simulink library "adrcLibrary"  (R2021a)
settings: Solver=VariableStepAuto  StartTime=0.0  StopTime=10.0  RelTol=1e-3
undefined symbols (not defined in the file or in its folder): DiscIntNeverNeededParam, r0
settings Model: Creator=onqi  LastModifiedBy=onqi

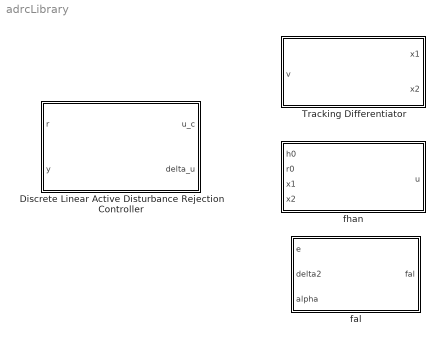
== system adrcLibrary ==
  Discrete Linear Active Disturbance Rejection Controller : Subsystem  Variant=on  VariantControl=Choice  mask(Linear Active Disturbance Rejection Control){order=1, b0=1, w_cl=1, k_eso=1, eso_init=[0;0], m_lim=[-inf, inf], r_lim=[-inf, inf], halfgain_ctrl=off, halfgain_obsv=off, inc_form=on, SampleTime=-1}
      mask prompts: order "First- or second-order ADRC"; b0 "Gain parameter b0"; w_cl "Desired closed-loop bandwidth w_cl [rad/s]"; k_eso "Relational observer bandwidth k_eso"; eso_init "Initial state of extended state observer"; m_lim "Magnitude limit of controller [lo, hi]"; r_lim "Rate limit of controller [lo, hi]"; halfgain_ctrl "Toggle half-gain tuning for controller"; halfgain_obsv "Toggle half-gain tuning for observer"; inc_form "Incremental form of ADRC"; SampleTime "Simulink:blkprm_prompts:AllBlksSampleTime"
      mask help:
      | Linear Active Disturbance Rejection Control block implementing the algorithms described in
      |
      | - Practical Active Disturbance Rejection Control: Bumpless Transfer, Rate Limitation and Incremental Algorithm, Gernot Herbst
      | - Half-Gain Tuning for Active Disturbance Rejection Control, Herbst et al.
      mask init:
      | ADRC_INC_FORM = inc_form;
      | 
      | if order == 1
      |     Ad = [[1, SampleTime];[0, 1]];
      |     Bd = [b0 * SampleTime; 0];
      |     Cd = [1, 0];
      |     Dd = 0;
      |     % Controller parameters for closed-loop dynamics
      |     t_settle = 4 / w_cl;
      |     sCL = -4 / t_settle;
      |     Kp = -2 * sCL;
      |     % Observer dynamics
      |     sESO = k_eso * sCL;
      |     zESO = exp(sESO * SampleTime);
      | 
      |     % Observer gains resulting in common-location observer poles
      |     L = [1 - zESO^2; (1 / SampleTime) * (1 - zESO)^2];
      | 
      |     % Controller gains
      |     w = [Kp / b0; 1 / b0];
      | 
      | elseif order == 2
      |     Ad = [[1, SampleTime, (SampleTime^2) / 2]; [0, 1, SampleTime]; [0, 0, 1]];
      |     Bd = [b0 * (SampleTime^2) / 2; b0 * SampleTime; 0];
      |     Cd = [1, 0, 0];
      |     Dd = 0;
      | 
      |     % Controller parameters for closed-loop dynamics
      |     t_settle = 6 / w_cl;
      |     sCL = -6 / t_settle;
      |     Kp = sCL^2;
      |     Kd = -2 * sCL;
      | 
      |     % Observer dynamics
      |     sESO = k_eso * sCL;
      |     zESO = exp(sESO * SampleTime);
      | 
      |     % Observer gains resulting in common-location observer poles
      |     L = [1 - (zESO)^3; (3 / (2 * SampleTime)) * (1 - zESO)^2 * (1 + zESO); 
      |         (1 / SampleTime^2) * (1 - zESO)^3];
      | 
      |     % Controller gains
      |     w = [Kp / b0; Kd / b0; 1 / b0];
      | end
      | 
      | if halfgain_obsv
      |     L = L/2;
      | end
      | 
      | if halfgain_ctrl
      |     w = w/2;
      | end
      | 
      | % One-step update equation implementing linear ESO
      | A_ESO = Ad - L * Cd * Ad;
      | B_ESO = Bd - L * Cd * Bd;
      | C_ESO = Cd;
      | 
      | L_ESO = L;
      settings: CopyFcn=set_param(gcbh,'LinkStatus','none');
      mask TypeOptions order: 1 | 2
      mask TypeOptions SampleTime: r/SampleTime
      mask DialogControl SampleTime Prompt: Sample time (-1 for inherited):
      mask Display:
      | disp('Discrete Linear\nADRC');
      | 
      | port_label('output', 1, 'u[k]', 'texmode', 'on');
      | port_label('input', 2, 'y[k-1]', 'texmode', 'on');
      | port_label('input', 1, 'r[k]', 'texmode', 'on');
      | 
      | if ADRC_INC_FORM == 1
      |     port_label('output', 2, '\Deltau', 'texmode', 'on');
      | end
  Tracking Differentiator : Subsystem  SystemSampleTime=SystemSampleTime  mask{r0=50, h0=10, SystemSampleTime=-1}
      mask prompts: r0 "Tracking speed r0"; h0 "Tracking smoothness h0"; SystemSampleTime "Simulink:blkprm_prompts:AllBlksSampleTime"
      mask init:
      | h = str2num(get_param(gcs,'FixedStep'));
      mask TypeOptions SystemSampleTime: SystemSampleTime
      mask DialogControl SystemSampleTime Prompt: Sample time (-1 for inherited):
      mask Display:
      | disp('Tracking Differentiator')
      | port_label('input', 1, '\vee', 'texmode', 'on');
      | port_label('output', 1, 'x_1', 'texmode', 'on');
      | port_label('output', 2, '\Deltax_1', 'texmode', 'on');
  fal : Subsystem
      mask Display:
      | disp('fal(e, \alpha, \delta)', 'texmode', 'on')
      | port_label('input', 1, 'e', 'texmode', 'on');
      | port_label('output', 1, 'fal', 'texmode', 'on');
      | port_label('input', 2, '\delta', 'texmode', 'on');
      | port_label('input', 3, '\alpha', 'texmode', 'on');
  fhan : Subsystem
      mask Display:
      | disp('fhan(x_1, x_2, r, h)', 'texmode', 'on')
      | port_label('input', 1, 'h_0', 'texmode', 'on');
      | port_label('input', 2, 'r_0', 'texmode', 'on');
      | port_label('input', 3, 'x_1', 'texmode', 'on');
      | port_label('input', 4, 'x_2', 'texmode', 'on');
      | 
      | port_label('output', 1, 'f_{han}', 'texmode', 'on');

== system adrcLibrary/Discrete Linear Active Disturbance Rejection Controller ==
  r : Inport  SampleTime=SampleTime
  y : Inport  Port=2
  Incremental Form : Subsystem  VariantControl=inc_form == 1
  Non-Incremental Form : Subsystem  VariantControl=inc_form == 0
  u_c : Outport
  delta_u : Outport  Port=2

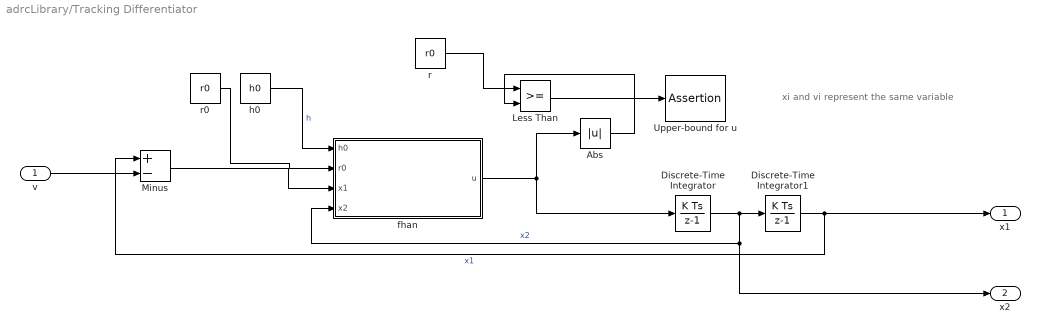
== system adrcLibrary/Tracking Differentiator ==
  note: xi and vi represent the same variable
  v : Inport
  Abs : Abs
  Discrete-Time Integrator : DiscreteIntegrator  SampleTime=-1  ICPrevOutput=DiscIntNeverNeededParam  ICPrevScaledInput=DiscIntNeverNeededParam
  Discrete-Time Integrator1 : DiscreteIntegrator  SampleTime=-1  ICPrevOutput=DiscIntNeverNeededParam  ICPrevScaledInput=DiscIntNeverNeededParam
  Less Than : RelationalOperator  OutDataTypeStr=boolean  RndMeth=Simplest
  Minus : Sum  Inputs=+-
  Upper-bound for u : Assertion
  fhan : Subsystem
  h0 : Constant  Value=h0  SampleTime=-1
  r : Constant  Value=r0  SampleTime=-1
  r0 : Constant  Value=r0  SampleTime=-1
  x1 : Outport
  x2 : Outport  Port=2
  wires:
  Abs/1 -> Less Than/2
  Less Than/1 -> Upper-bound for u/1
  Discrete-Time Integrator1/1 -> x1/1, Minus/1  "x1"
  Discrete-Time Integrator/1 -> fhan/4(x2), x2/1, Discrete-Time Integrator1/1  "x2"
  v/1 -> Minus/2
  r/1 -> Less Than/1
  fhan/1(u) -> Discrete-Time Integrator/1, Abs/1
  h0/1 -> fhan/1(h0)  "h"
  r0/1 -> fhan/2(r0)
  Minus/1 -> fhan/3(x1)

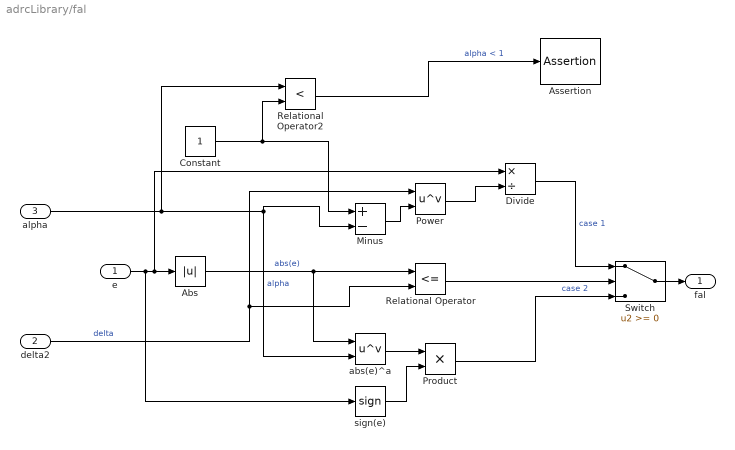
== system adrcLibrary/fal ==
  e : Inport
  delta2 : Inport  Port=2
  alpha : Inport  Port=3
  Abs : Abs
  Assertion : Assertion
  Constant : Constant
  Divide : Product  Inputs=*/
  Minus : Sum  Inputs=+-
  Power : Math  Operator=pow  SaturateOnIntegerOverflow=on
  Product : Product
  Relational Operator : RelationalOperator  Operator=<=  OutDataTypeStr=boolean  RndMeth=Simplest
  Relational Operator2 : RelationalOperator  Operator=<  OutDataTypeStr=boolean  RndMeth=Simplest
  Switch : Switch
  abs(e)^a : Math  Operator=pow  SaturateOnIntegerOverflow=on
  sign(e) : Signum
  fal : Outport
  wires:
  sign(e)/1 -> Product/2
  Switch/1 -> fal/1
  Relational Operator/1 -> Switch/2
  Abs/1 -> abs(e)^a/1, Relational Operator/1  "abs(e)"
  Power/1 -> Divide/2
  alpha/1 -> Relational Operator2/1, Minus/2, abs(e)^a/2  "alpha"
  Minus/1 -> Power/2
  e/1 -> sign(e)/1, Divide/1, Abs/1
  abs(e)^a/1 -> Product/1
  Product/1 -> Switch/3  "case 2"
  Divide/1 -> Switch/1  "case 1"
  delta2/1 -> Relational Operator/2, Power/1  "delta"
  Constant/1 -> Relational Operator2/2, Minus/1
  Relational Operator2/1 -> Assertion/1  "alpha < 1"

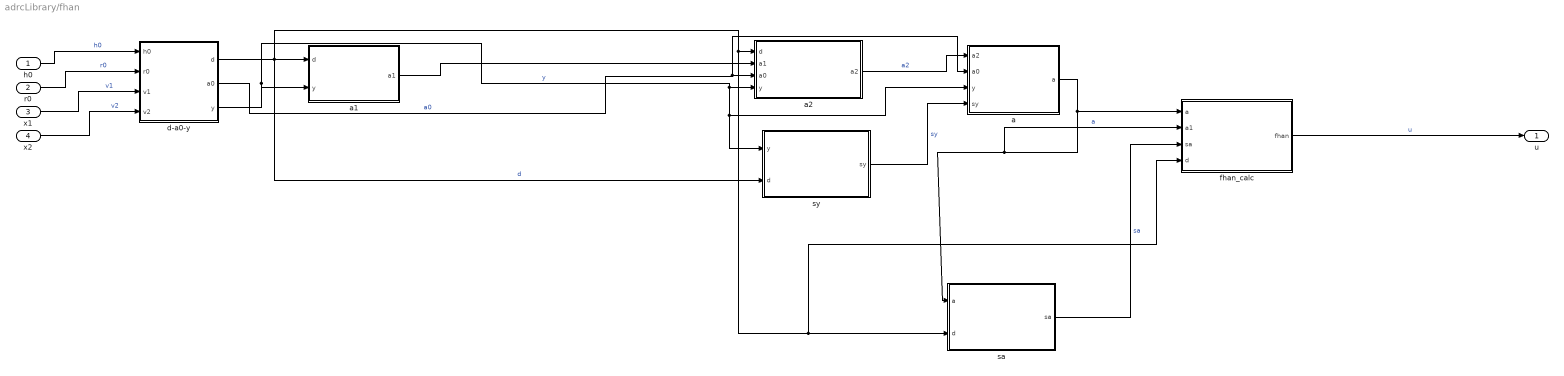
== system adrcLibrary/fhan ==
  h0 : Inport
  r0 : Inport  Port=2
  x1 : Inport  Port=3
  x2 : Inport  Port=4
  a : Subsystem
  a1 : Subsystem
  a2 : Subsystem
  d-a0-y : Subsystem
  fhan_calc : Subsystem
  sa : Subsystem
  sy : Subsystem
  u : Outport
  wires:
  h0/1 -> d-a0-y/1(h0)  "h0"
  r0/1 -> d-a0-y/2(r0)  "r0"
  x1/1 -> d-a0-y/3(v1)  "v1"
  x2/1 -> d-a0-y/4(v2)  "v2"
  d-a0-y/1(d) -> sy/2(d), a1/1(d), fhan_calc/4(d), sa/2(d), a2/1(d)  "d"
  d-a0-y/3(y) -> a/3(y), sy/1(y), a2/4(y), a1/2(y)  "y"
  a1/1(a1) -> a2/2(a1)
  d-a0-y/2(a0) -> a/2(a0), a2/3(a0)  "a0"
  a2/1(a2) -> a/1(a2)  "a2"
  sy/1(sy) -> a/4(sy)  "sy"
  a/1(a) -> sa/1(a), fhan_calc/2(a1), fhan_calc/1(a)  "a"
  sa/1(sa) -> fhan_calc/3(sa)  "sa"
  fhan_calc/1(fhan) -> u/1  "u"

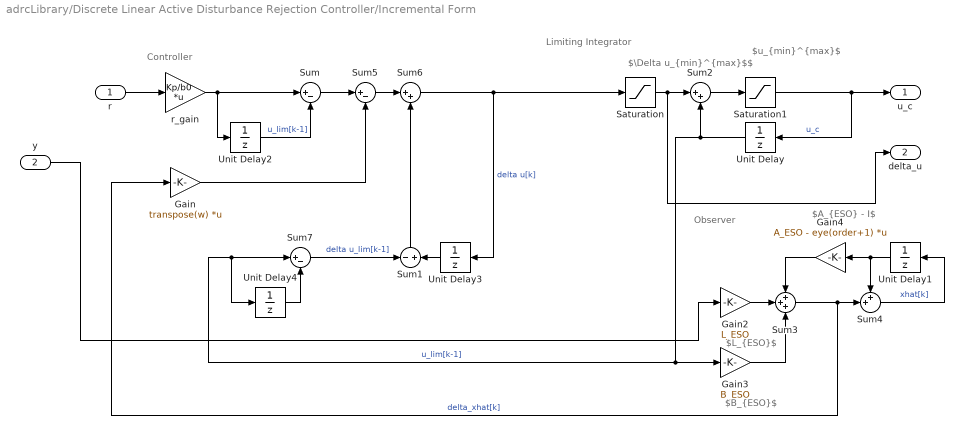
== system adrcLibrary/Discrete Linear Active Disturbance Rejection Controller/Incremental Form ==
  note: Controller
  note: $\Delta u_{min}^{max}$$
  note: $u_{min}^{max}$
  note: $L_{ESO}$
  note: $B_{ESO}$
  note: $A_{ESO} - I$
  note: Limiting
      | 	Integrator
  note: Observer
  r : Inport  SampleTime=SampleTime
  y : Inport  Port=2
  Gain : Gain  Gain=transpose(w)  Multiplication=Matrix(K*u) (u vector)
  Gain2 : Gain  Gain=L_ESO
  Gain3 : Gain  Gain=B_ESO
  Gain4 : Gain  Gain=A_ESO - eye(order+1)  Multiplication=Matrix(K*u) (u vector)
  Saturation : Saturate  UpperLimit=r_lim(2)  LowerLimit=r_lim(1)
  Saturation1 : Saturate  UpperLimit=m_lim(2)  LowerLimit=m_lim(1)
  Sum : Sum  Inputs=|+-
  Sum1 : Sum  Inputs=-+
  Sum2 : Sum  Inputs=|++
  Sum3 : Sum  Inputs=+++
  Sum4 : Sum  Inputs=++|
  Sum5 : Sum  Inputs=|+-
  Sum6 : Sum  Inputs=|++
  Sum7 : Sum  Inputs=|+-
  Unit Delay{,1..4} (5 alike) : UnitDelay  SampleTime=-1  HasFrameUpgradeWarning=on
  r_gain : Gain  Gain=Kp/b0  Multiplication=Matrix(K*u) (u vector)
  u_c : Outport
  delta_u : Outport  Port=2
  wires:
  Unit Delay1/1 -> Sum4/1, Gain4/1
  Sum2/1 -> Saturation1/1
  Gain4/1 -> Sum3/1
  Gain3/1 -> Sum3/3
  y/1 -> Gain2/1
  Sum6/1 -> Unit Delay3/1, Saturation/1  "delta u[k]"
  Saturation1/1 -> u_c/1, Unit Delay/1  "u_c"
  Unit Delay/1 -> Gain3/1, Unit Delay4/1, Sum7/1, Sum2/2  "u_lim[k-1]"
  Saturation/1 -> delta_u/1, Sum2/1
  r_gain/1 -> Unit Delay2/1, Sum/1
  r/1 -> r_gain/1
  Gain2/1 -> Sum3/2
  Sum4/1 -> Unit Delay1/1  "xhat[k]"
  Sum3/1 -> Gain/1, Sum4/2  "delta_xhat[k]"
  Sum/1 -> Sum5/1
  Sum5/1 -> Sum6/1
  Unit Delay2/1 -> Sum/2  "u_lim[k-1]"
  Gain/1 -> Sum5/2
  Unit Delay3/1 -> Sum1/2
  Sum1/1 -> Sum6/2
  Sum7/1 -> Sum1/1  "delta u_lim[k-1]"
  Unit Delay4/1 -> Sum7/2

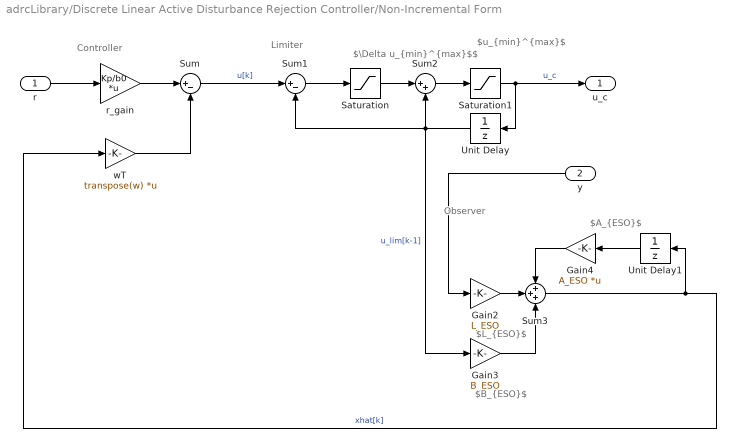
== system adrcLibrary/Discrete Linear Active Disturbance Rejection Controller/Non-Incremental Form ==
  note: Controller
  note: $\Delta u_{min}^{max}$$
  note: $u_{min}^{max}$
  note: $L_{ESO}$
  note: $B_{ESO}$
  note: $A_{ESO}$
  note: Limiter
  note: Observer
  r : Inport  SampleTime=SampleTime
  y : Inport  Port=2
  Gain2 : Gain  Gain=L_ESO
  Gain3 : Gain  Gain=B_ESO
  Gain4 : Gain  Gain=A_ESO  Multiplication=Matrix(K*u) (u vector)
  Saturation : Saturate  UpperLimit=r_lim(2)  LowerLimit=r_lim(1)
  Saturation1 : Saturate  UpperLimit=m_lim(2)  LowerLimit=m_lim(1)
  Sum : Sum  Inputs=|+-
  Sum1 : Sum  Inputs=|+-
  Sum2 : Sum  Inputs=|++
  Sum3 : Sum  Inputs=+++
  Unit Delay : UnitDelay  SampleTime=-1  HasFrameUpgradeWarning=on
  Unit Delay1 : UnitDelay  SampleTime=-1  HasFrameUpgradeWarning=on
  r_gain : Gain  Gain=Kp/b0  Multiplication=Matrix(K*u) (u vector)
  wT : Gain  Gain=transpose(w)  Multiplication=Matrix(K*u) (u vector)
  u_c : Outport
  wires:
  Unit Delay1/1 -> Gain4/1
  wT/1 -> Sum/2
  Sum2/1 -> Saturation1/1
  Gain4/1 -> Sum3/1
  Gain3/1 -> Sum3/3
  y/1 -> Gain2/1
  Sum1/1 -> Saturation/1
  Saturation1/1 -> u_c/1, Unit Delay/1  "u_c"
  Unit Delay/1 -> Gain3/1, Sum2/2, Sum1/2  "u_lim[k-1]"
  Saturation/1 -> Sum2/1
  r_gain/1 -> Sum/1
  r/1 -> r_gain/1
  Sum/1 -> Sum1/1  "u[k]"
  Sum3/1 -> wT/1, Unit Delay1/1  "xhat[k]"
  Gain2/1 -> Sum3/2

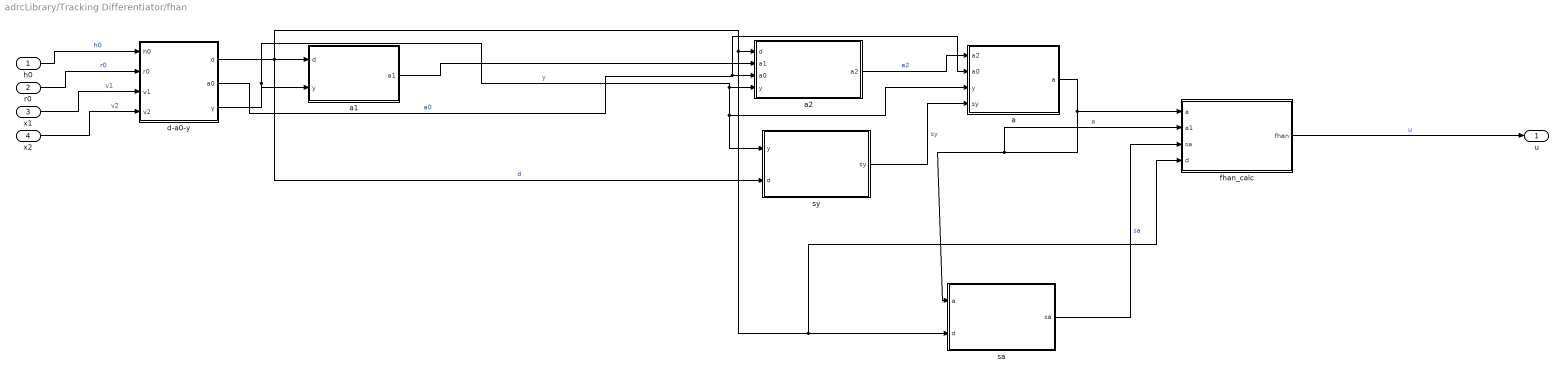
== system adrcLibrary/Tracking Differentiator/fhan ==
  h0 : Inport
  r0 : Inport  Port=2
  x1 : Inport  Port=3
  x2 : Inport  Port=4
  a : Subsystem
  a1 : Subsystem
  a2 : Subsystem
  d-a0-y : Subsystem
  fhan_calc : Subsystem
  sa : Subsystem
  sy : Subsystem
  u : Outport
  wires:
  h0/1 -> d-a0-y/1(h0)  "h0"
  r0/1 -> d-a0-y/2(r0)  "r0"
  x1/1 -> d-a0-y/3(v1)  "v1"
  x2/1 -> d-a0-y/4(v2)  "v2"
  d-a0-y/1(d) -> sy/2(d), a1/1(d), fhan_calc/4(d), sa/2(d), a2/1(d)  "d"
  d-a0-y/3(y) -> a/3(y), sy/1(y), a2/4(y), a1/2(y)  "y"
  a1/1(a1) -> a2/2(a1)
  d-a0-y/2(a0) -> a/2(a0), a2/3(a0)  "a0"
  a2/1(a2) -> a/1(a2)  "a2"
  sy/1(sy) -> a/4(sy)  "sy"
  a/1(a) -> sa/1(a), fhan_calc/2(a1), fhan_calc/1(a)  "a"
  sa/1(sa) -> fhan_calc/3(sa)  "sa"
  fhan_calc/1(fhan) -> u/1  "u"

== system adrcLibrary/fhan/a ==
  a2 : Inport
  a0 : Inport  Port=2
  y : Inport  Port=3
  sy : Inport  Port=4
  Add : Sum  Inputs=++-
  Plus : Sum
  Product : Product
  a : Outport
  wires:
  y/1 -> Add/2
  a0/1 -> Add/1
  Plus/1 -> a/1  "a"
  a2/1 -> Plus/2, Add/3
  Product/1 -> Plus/1
  sy/1 -> Product/2
  Add/1 -> Product/1

== system adrcLibrary/fhan/a1 ==
  d : Inport
  y : Inport  Port=2
  Abs : Abs
  Add : Sum
  Gain : Gain  Gain=8
  Product : Product
  Sqrt : Sqrt  SaturateOnIntegerOverflow=on
  a1 : Outport
  wires:
  Product/1 -> Sqrt/1
  Sqrt/1 -> a1/1  "a1"
  y/1 -> Abs/1
  d/1 -> Product/1, Add/1
  Add/1 -> Product/2
  Abs/1 -> Gain/1
  Gain/1 -> Add/2  "8|y|"

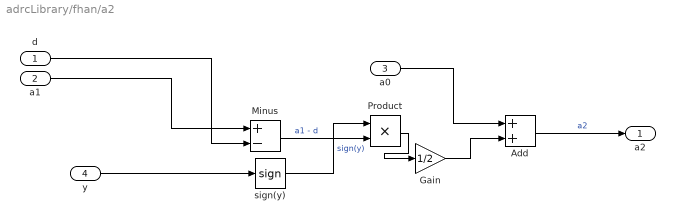
== system adrcLibrary/fhan/a2 ==
  d : Inport
  a1 : Inport  Port=2
  a0 : Inport  Port=3
  y : Inport  Port=4
  Add : Sum
  Gain : Gain  Gain=1/2
  Minus : Sum  Inputs=+-
  Product : Product
  sign(y) : Signum
  a2 : Outport
  wires:
  sign(y)/1 -> Product/1  "sign(y)"
  Minus/1 -> Product/2  "a1 - d"
  Product/1 -> Gain/1
  y/1 -> sign(y)/1
  a0/1 -> Add/1
  d/1 -> Minus/2
  Add/1 -> a2/1  "a2"
  a1/1 -> Minus/1
  Gain/1 -> Add/2

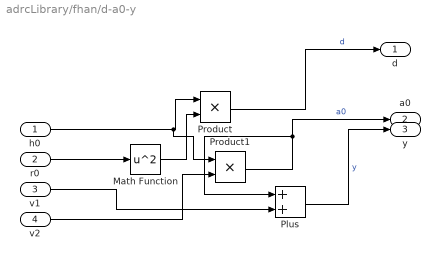
== system adrcLibrary/fhan/d-a0-y ==
  h0 : Inport
  r0 : Inport  Port=2
  v1 : Inport  Port=3
  v2 : Inport  Port=4
  Math Function : Math  Operator=square  SaturateOnIntegerOverflow=on
  Plus : Sum
  Product : Product
  Product1 : Product
  d : Outport
  a0 : Outport  Port=2
  y : Outport  Port=3
  wires:
  Math Function/1 -> Product/2
  v1/1 -> Plus/2
  Plus/1 -> y/1  "y"
  r0/1 -> Math Function/1
  Product1/1 -> a0/1, Plus/1  "a0"
  v2/1 -> Product1/2
  Product/1 -> d/1  "d"
  h0/1 -> Product1/1, Product/1

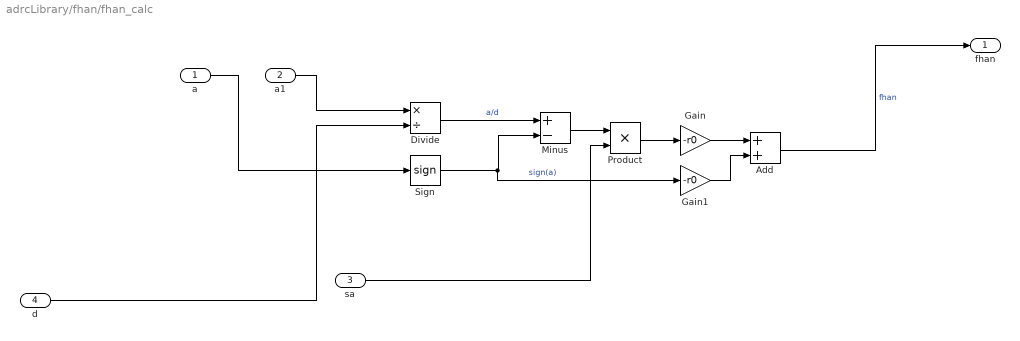
== system adrcLibrary/fhan/fhan_calc ==
  a : Inport
  a1 : Inport  Port=2
  sa : Inport  Port=3
  d : Inport  Port=4
  Add : Sum
  Divide : Product  Inputs=*/
  Gain : Gain  Gain=-r0
  Gain1 : Gain  Gain=-r0
  Minus : Sum  Inputs=+-
  Product : Product
  Sign : Signum
  fhan : Outport
  wires:
  sa/1 -> Product/2
  Minus/1 -> Product/1
  Gain/1 -> Add/1
  Divide/1 -> Minus/1  "a/d"
  a/1 -> Sign/1
  Add/1 -> fhan/1  "fhan"
  a1/1 -> Divide/1
  Gain1/1 -> Add/2
  d/1 -> Divide/2
  Product/1 -> Gain/1
  Sign/1 -> Gain1/1, Minus/2  "sign(a)"

== system adrcLibrary/fhan/sa ==
  a : Inport
  d : Inport  Port=2
  Gain : Gain  Gain=1/2
  Minus : Sum  Inputs=+-
  Minus1 : Sum  Inputs=+-
  Plus : Sum
  Sign1 : Signum
  Sign2 : Signum
  sa : Outport
  wires:
  Sign1/1 -> Minus1/1
  Plus/1 -> Sign1/1
  a/1 -> Minus/1, Plus/1
  Sign2/1 -> Minus1/2
  Minus/1 -> Sign2/1
  Minus1/1 -> Gain/1
  d/1 -> Minus/2, Plus/2
  Gain/1 -> sa/1  "s"

== system adrcLibrary/fhan/sy ==
  y : Inport
  d : Inport  Port=2
  Gain : Gain  Gain=1/2
  Minus : Sum  Inputs=+-
  Minus1 : Sum  Inputs=+-
  Plus : Sum
  Sign1 : Signum
  Sign2 : Signum
  sy : Outport
  wires:
  Sign1/1 -> Minus1/1
  Plus/1 -> Sign1/1
  y/1 -> Minus/1, Plus/1
  Sign2/1 -> Minus1/2
  Minus/1 -> Sign2/1
  Minus1/1 -> Gain/1
  d/1 -> Minus/2, Plus/2
  Gain/1 -> sy/1  "s"

== system adrcLibrary/Tracking Differentiator/fhan/a ==
  a2 : Inport
  a0 : Inport  Port=2
  y : Inport  Port=3
  sy : Inport  Port=4
  Add : Sum  Inputs=++-
  Plus : Sum
  Product : Product
  a : Outport
  wires:
  y/1 -> Add/2
  a0/1 -> Add/1
  Plus/1 -> a/1  "a"
  a2/1 -> Plus/2, Add/3
  Product/1 -> Plus/1
  sy/1 -> Product/2
  Add/1 -> Product/1

== system adrcLibrary/Tracking Differentiator/fhan/a1 ==
  d : Inport
  y : Inport  Port=2
  Abs : Abs
  Add : Sum
  Gain : Gain  Gain=8
  Product : Product
  Sqrt : Sqrt  SaturateOnIntegerOverflow=on
  a1 : Outport
  wires:
  Product/1 -> Sqrt/1
  Sqrt/1 -> a1/1  "a1"
  y/1 -> Abs/1
  d/1 -> Product/1, Add/1
  Add/1 -> Product/2
  Abs/1 -> Gain/1
  Gain/1 -> Add/2  "8|y|"

== system adrcLibrary/Tracking Differentiator/fhan/a2 ==
  d : Inport
  a1 : Inport  Port=2
  a0 : Inport  Port=3
  y : Inport  Port=4
  Add : Sum
  Gain : Gain  Gain=1/2
  Minus : Sum  Inputs=+-
  Product : Product
  sign(y) : Signum
  a2 : Outport
  wires:
  sign(y)/1 -> Product/1  "sign(y)"
  Minus/1 -> Product/2  "a1 - d"
  Product/1 -> Gain/1
  y/1 -> sign(y)/1
  a0/1 -> Add/1
  d/1 -> Minus/2
  Add/1 -> a2/1  "a2"
  a1/1 -> Minus/1
  Gain/1 -> Add/2

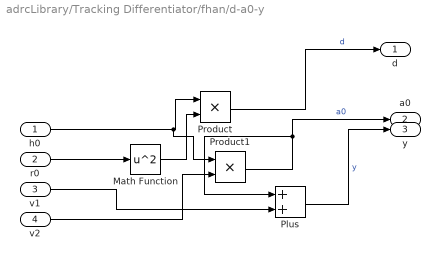
== system adrcLibrary/Tracking Differentiator/fhan/d-a0-y ==
  h0 : Inport
  r0 : Inport  Port=2
  v1 : Inport  Port=3
  v2 : Inport  Port=4
  Math Function : Math  Operator=square  SaturateOnIntegerOverflow=on
  Plus : Sum
  Product : Product
  Product1 : Product
  d : Outport
  a0 : Outport  Port=2
  y : Outport  Port=3
  wires:
  Math Function/1 -> Product/2
  v1/1 -> Plus/2
  Plus/1 -> y/1  "y"
  r0/1 -> Math Function/1
  Product1/1 -> a0/1, Plus/1  "a0"
  v2/1 -> Product1/2
  Product/1 -> d/1  "d"
  h0/1 -> Product1/1, Product/1

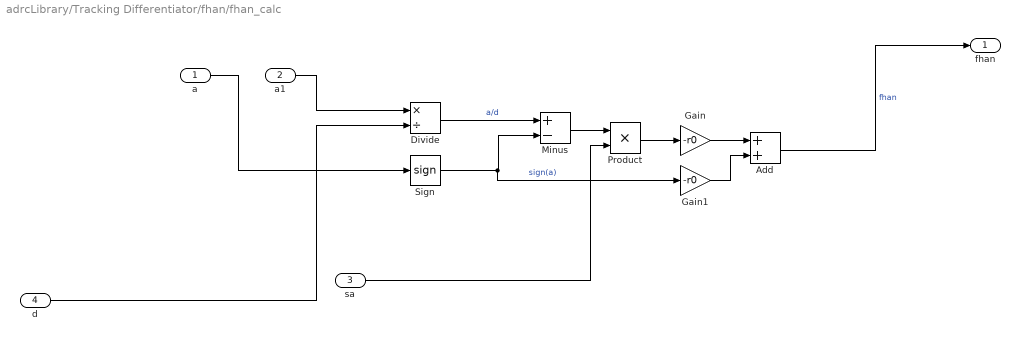
== system adrcLibrary/Tracking Differentiator/fhan/fhan_calc ==
  a : Inport
  a1 : Inport  Port=2
  sa : Inport  Port=3
  d : Inport  Port=4
  Add : Sum
  Divide : Product  Inputs=*/
  Gain : Gain  Gain=-r0
  Gain1 : Gain  Gain=-r0
  Minus : Sum  Inputs=+-
  Product : Product
  Sign : Signum
  fhan : Outport
  wires:
  sa/1 -> Product/2
  Minus/1 -> Product/1
  Gain/1 -> Add/1
  Divide/1 -> Minus/1  "a/d"
  a/1 -> Sign/1
  Add/1 -> fhan/1  "fhan"
  a1/1 -> Divide/1
  Gain1/1 -> Add/2
  d/1 -> Divide/2
  Product/1 -> Gain/1
  Sign/1 -> Gain1/1, Minus/2  "sign(a)"

== system adrcLibrary/Tracking Differentiator/fhan/sa ==
  a : Inport
  d : Inport  Port=2
  Gain : Gain  Gain=1/2
  Minus : Sum  Inputs=+-
  Minus1 : Sum  Inputs=+-
  Plus : Sum
  Sign1 : Signum
  Sign2 : Signum
  sa : Outport
  wires:
  Sign1/1 -> Minus1/1
  Plus/1 -> Sign1/1
  a/1 -> Minus/1, Plus/1
  Sign2/1 -> Minus1/2
  Minus/1 -> Sign2/1
  Minus1/1 -> Gain/1
  d/1 -> Minus/2, Plus/2
  Gain/1 -> sa/1  "s"

== system adrcLibrary/Tracking Differentiator/fhan/sy ==
  y : Inport
  d : Inport  Port=2
  Gain : Gain  Gain=1/2
  Minus : Sum  Inputs=+-
  Minus1 : Sum  Inputs=+-
  Plus : Sum
  Sign1 : Signum
  Sign2 : Signum
  sy : Outport
  wires:
  Sign1/1 -> Minus1/1
  Plus/1 -> Sign1/1
  y/1 -> Minus/1, Plus/1
  Sign2/1 -> Minus1/2
  Minus/1 -> Sign2/1
  Minus1/1 -> Gain/1
  d/1 -> Minus/2, Plus/2
  Gain/1 -> sy/1  "s"
